simulink model "robot_adaptive_control"  (Simulink 7.2)
settings: Solver=ode45  StartTime=0.0  StopTime=20  RelTol=1e-3
libraries: dspmtrx3 x9, simulink x3
settings Model: Creator=GILL  LastModifiedBy=Dany
settings ConfigComp: Description=Design Verifier Custom Configuration Component  DVMaxProcessTime=600  DVDisplayUnsatisfiableObjectives=on  DVModelCoverageObjectives=MCDC  DVMaxTestCaseSteps=500  DVTestSuiteOptimization=CombinedObjectives  DVSaveHarnessModel=on  DVSaveReport=on

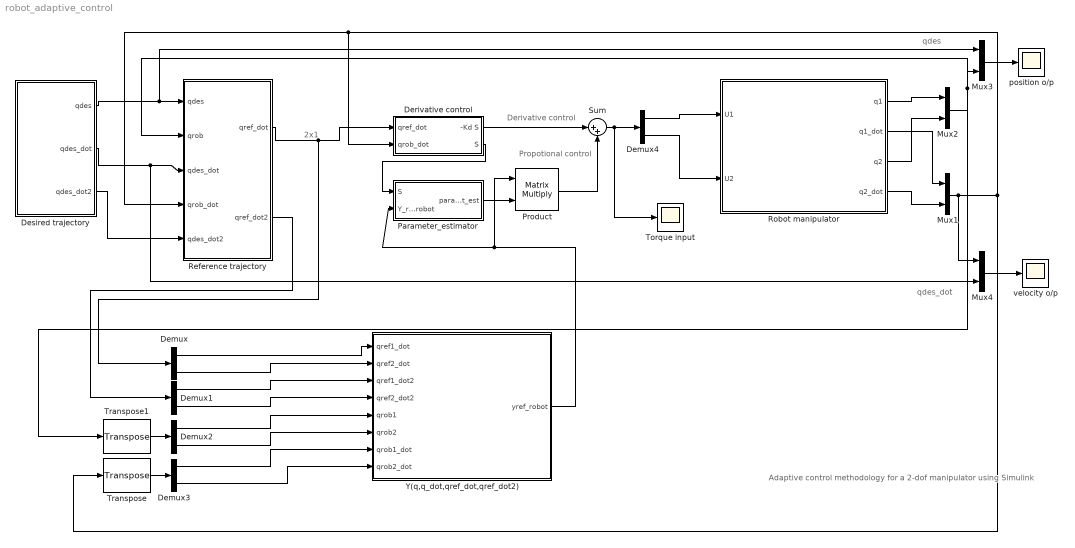
== system robot_adaptive_control ==
  note: 2x1
  note: qdes_dot
  note: qdes
  note: Propotional control
  note: Derivative control
  note: Adaptive control methodology for
      | a 2-dof manipulator using Simulink
  Demux{,1..4} (5 alike) : Demux  Outputs=2
  Derivative control : Subsystem
  Desired trajectory : Subsystem
  Mux{1..4} (4 alike) : Mux  Inputs=2
  Parameter_estimator : Subsystem
  Product : Product  Multiplication=Matrix(*)  OutDataType=fixdt(1, 16)  OutScaling=2^0  RndMeth=Zero
  Reference trajectory : Subsystem
  "Robot manipulator " : Subsystem
  Sum : Sum  Inputs=|++
  "Torque input " : Scope
      settings: YMin=-1.6  YMax=0.3  SaveName=ScopeData2
  Transpose : dspmtrx3/Transpose  SystemSampleTime=-1  Hermitian=off  overflowFlag=off
  Transpose1 : dspmtrx3/Transpose  SystemSampleTime=-1  Hermitian=off  overflowFlag=off
  Y(q,q_dot,qref_dot,qref_dot2) : Stateflow chart
  "position o/p " : Scope
      settings: YMin=-1.6  YMax=0.3
  velocity o/p : Scope
      settings: YMin=-1.6  YMax=0.3
  wires:
  Desired trajectory/1(qdes) -> Reference trajectory/1(qdes), Mux3/1
  Desired trajectory/2(qdes_dot) -> Reference trajectory/3(qdes_dot), Mux4/2
  Desired trajectory/3(qdes_dot2) -> Reference trajectory/5(qdes_dot2)
  Reference trajectory/1(qref_dot) -> Derivative control/1(qref_dot), Demux/1
  Demux/1 -> Y(q,q_dot,qref_dot,qref_dot2)/1(qref1_dot)
  Demux/2 -> Y(q,q_dot,qref_dot,qref_dot2)/2(qref2_dot)
  Demux1/1 -> Y(q,q_dot,qref_dot,qref_dot2)/3(qref1_dot2)
  Demux1/2 -> Y(q,q_dot,qref_dot,qref_dot2)/4(qref2_dot2)
  Demux2/1 -> Y(q,q_dot,qref_dot,qref_dot2)/5(qrob1)
  Demux2/2 -> Y(q,q_dot,qref_dot,qref_dot2)/6(qrob2)
  Demux3/1 -> Y(q,q_dot,qref_dot,qref_dot2)/7(qrob1_dot)
  Demux3/2 -> Y(q,q_dot,qref_dot,qref_dot2)/8(qrob2_dot)
  Reference trajectory/2(qref_dot2) -> Demux1/1
  Derivative control/1(-Kd S) -> Sum/1
  Derivative control/2(S) -> Parameter_estimator/1(S)
  Product/1 -> Sum/2
  Sum/1 -> Demux4/1, "Torque input "/1
  Mux1/1 -> Mux4/1, Transpose/1, Derivative control/2(qrob_dot), Reference trajectory/4(qrob_dot)
  Mux2/1 -> Mux3/2, Transpose1/1, Reference trajectory/2(qrob)
  Transpose1/1 -> Demux2/1
  Transpose/1 -> Demux3/1
  Y(q,q_dot,qref_dot,qref_dot2)/1(yref_robot) -> Product/1, Parameter_estimator/2(Y_ref_robot)
  Parameter_estimator/1(paramt_est) -> Product/2
  Mux3/1 -> "position o/p "/1
  Mux4/1 -> velocity o/p/1
  Demux4/1 -> "Robot manipulator "/1(U1)
  Demux4/2 -> "Robot manipulator "/2(U2)
  "Robot manipulator "/1(q1) -> Mux2/1
  "Robot manipulator "/3(q2) -> Mux2/2
  "Robot manipulator "/2(q1_dot) -> Mux1/1
  "Robot manipulator "/4(q2_dot) -> Mux1/2

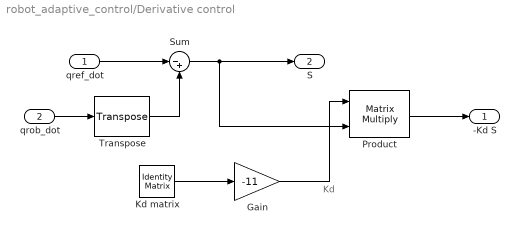
== system robot_adaptive_control/Derivative control ==
  note: Kd
  qref_dot : Inport
  qrob_dot : Inport  Port=2
  Gain : Gain  Gain=-11
  Kd matrix : dspmtrx3/Identity Matrix  Inherit=off  N=2  Ts=1  dataType=double  isSigned=on  wordLen=16  udDataType=sfix(16)  fracBitsMode=Best precision  numFracBits=15
  Product : Product  Multiplication=Matrix(*)  RndMeth=Zero
  Sum : Sum  Inputs=|-+
  Transpose : dspmtrx3/Transpose  SystemSampleTime=-1  Hermitian=off  overflowFlag=off
  -Kd S : Outport
  S : Outport  Port=2
  wires:
  qref_dot/1 -> Sum/1
  Sum/1 -> S/1, Product/2
  Kd matrix/1 -> Gain/1
  Product/1 -> -Kd S/1
  qrob_dot/1 -> Transpose/1
  Transpose/1 -> Sum/2
  Gain/1 -> Product/1

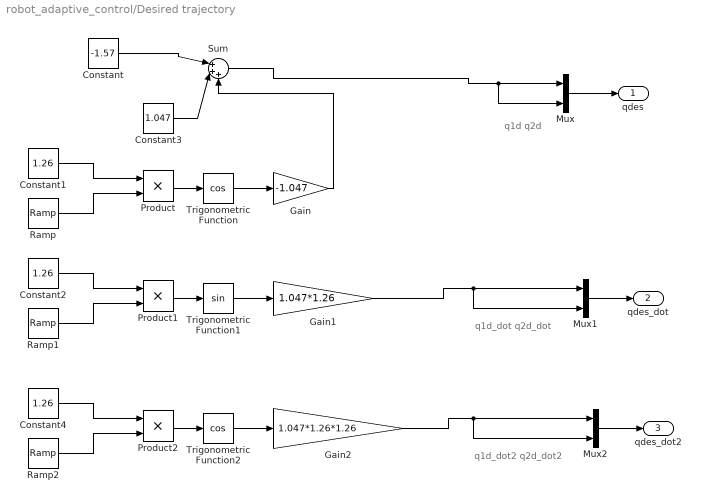
== system robot_adaptive_control/Desired trajectory ==
  note: q1d_dot
      | q2d_dot
  note: q1d
      | q2d
  note: q1d_dot2
      | q2d_dot2
  Constant : Constant  Value=-1.57
  Constant1 : Constant  Value=1.26
  Constant2 : Constant  Value=1.26
  Constant3 : Constant  Value=1.047
  Constant4 : Constant  Value=1.26
  Gain : Gain  Gain=-1.047
  Gain1 : Gain  Gain=1.047*1.26
  Gain2 : Gain  Gain=1.047*1.26*1.26
  Mux : Mux  Inputs=2
  Mux1 : Mux  Inputs=2
  Mux2 : Mux  Inputs=2
  Product : Product  RndMeth=Zero
  Product1 : Product  RndMeth=Zero
  Product2 : Product  RndMeth=Zero
  Ramp : simulink/Sources/Ramp  SystemSampleTime=-1  slope=1  start=0  X0=0
  Ramp1 : simulink/Sources/Ramp  SystemSampleTime=-1  slope=1  start=0  X0=0
  Ramp2 : simulink/Sources/Ramp  SystemSampleTime=-1  slope=1  start=0  X0=0
  Sum : Sum  Inputs=|+++
  Trigonometric Function : Trigonometry  Operator=cos
  Trigonometric Function1 : Trigonometry
  Trigonometric Function2 : Trigonometry  Operator=cos
  qdes : Outport
  qdes_dot : Outport  Port=2
  qdes_dot2 : Outport  Port=3
  wires:
  Constant/1 -> Sum/1
  Constant1/1 -> Product/1
  Constant3/1 -> Sum/2
  Ramp/1 -> Product/2
  Product/1 -> Trigonometric Function/1
  Trigonometric Function/1 -> Gain/1
  Gain/1 -> Sum/3
  Constant2/1 -> Product1/1
  Ramp1/1 -> Product1/2
  Product1/1 -> Trigonometric Function1/1
  Trigonometric Function1/1 -> Gain1/1
  Constant4/1 -> Product2/1
  Ramp2/1 -> Product2/2
  Product2/1 -> Trigonometric Function2/1
  Trigonometric Function2/1 -> Gain2/1
  Sum/1 -> Mux/1, Mux/2
  Mux/1 -> qdes/1
  Mux1/1 -> qdes_dot/1
  Gain1/1 -> Mux1/1, Mux1/2
  Mux2/1 -> qdes_dot2/1
  Gain2/1 -> Mux2/1, Mux2/2

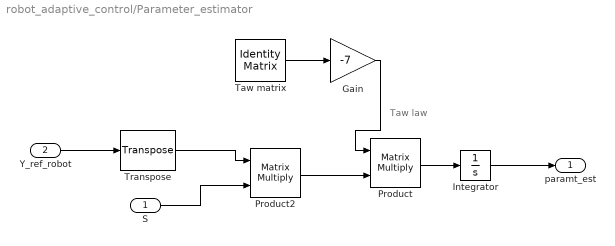
== system robot_adaptive_control/Parameter_estimator ==
  note: Taw law
  S : Inport  OutDataType=fixdt(1, 16)  OutScaling=2^0
  Y_ref_robot : Inport  Port=2  OutDataType=fixdt(1, 16)  OutScaling=2^0
  Gain : Gain  Gain=-7  ParameterDataType=fixdt(1, 16)  ParameterScaling=2^0  OutDataType=fixdt(1, 16)  OutScaling=2^0
  Integrator : Integrator
  Product : Product  Multiplication=Matrix(*)  OutDataType=fixdt(1, 16)  OutScaling=2^0  RndMeth=Zero
  Product2 : Product  Multiplication=Matrix(*)  OutDataType=fixdt(1, 16)  OutScaling=2^0  RndMeth=Zero
  Taw matrix : dspmtrx3/Identity Matrix  Inherit=off  N=5  Ts=1  dataType=double  isSigned=on  wordLen=16  udDataType=sfix(16)  fracBitsMode=Best precision  numFracBits=15
  Transpose : dspmtrx3/Transpose  SystemSampleTime=-1  Hermitian=off  overflowFlag=off
  paramt_est : Outport  OutDataType=fixdt(1, 16)  OutScaling=2^0
  wires:
  Product/1 -> Integrator/1
  Integrator/1 -> paramt_est/1
  Taw matrix/1 -> Gain/1
  Gain/1 -> Product/1
  Product2/1 -> Product/2
  Y_ref_robot/1 -> Transpose/1
  Transpose/1 -> Product2/1
  S/1 -> Product2/2

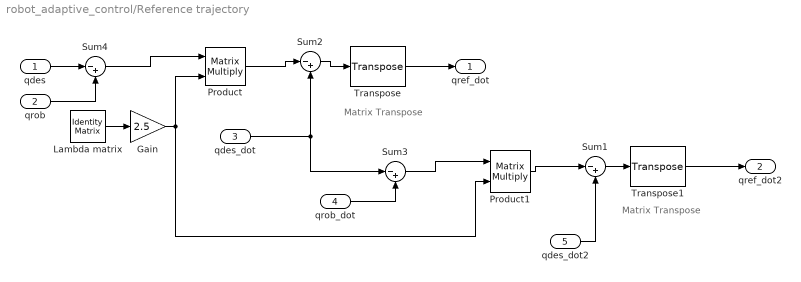
== system robot_adaptive_control/Reference trajectory ==
  note: Matrix Transpose
  note: Matrix Transpose
  qdes : Inport
  qrob : Inport  Port=2
  qdes_dot : Inport  Port=3
  qrob_dot : Inport  Port=4
  qdes_dot2 : Inport  Port=5
  Gain : Gain  Gain=2.5
  Lambda matrix : dspmtrx3/Identity Matrix  Inherit=off  N=2  Ts=1  dataType=double  isSigned=on  wordLen=16  udDataType=sfix(16)  fracBitsMode=Best precision  numFracBits=15
  Product : Product  Multiplication=Matrix(*)  RndMeth=Zero
  Product1 : Product  Multiplication=Matrix(*)  RndMeth=Zero
  Sum{1..4} (4 alike) : Sum  Inputs=|-+
  Transpose : dspmtrx3/Transpose  SystemSampleTime=-1  Hermitian=off  overflowFlag=off
  Transpose1 : dspmtrx3/Transpose  SystemSampleTime=-1  Hermitian=off  overflowFlag=off
  qref_dot : Outport
  qref_dot2 : Outport  Port=2
  wires:
  qdes/1 -> Sum4/1
  qrob/1 -> Sum4/2
  Sum4/1 -> Product/1
  Lambda matrix/1 -> Gain/1
  Gain/1 -> Product/2, Product1/2
  Product/1 -> Sum2/1
  qdes_dot/1 -> Sum2/2, Sum3/1
  qrob_dot/1 -> Sum3/2
  Sum3/1 -> Product1/1
  Product1/1 -> Sum1/1
  qdes_dot2/1 -> Sum1/2
  Transpose/1 -> qref_dot/1
  Sum2/1 -> Transpose/1
  Sum1/1 -> Transpose1/1
  Transpose1/1 -> qref_dot2/1

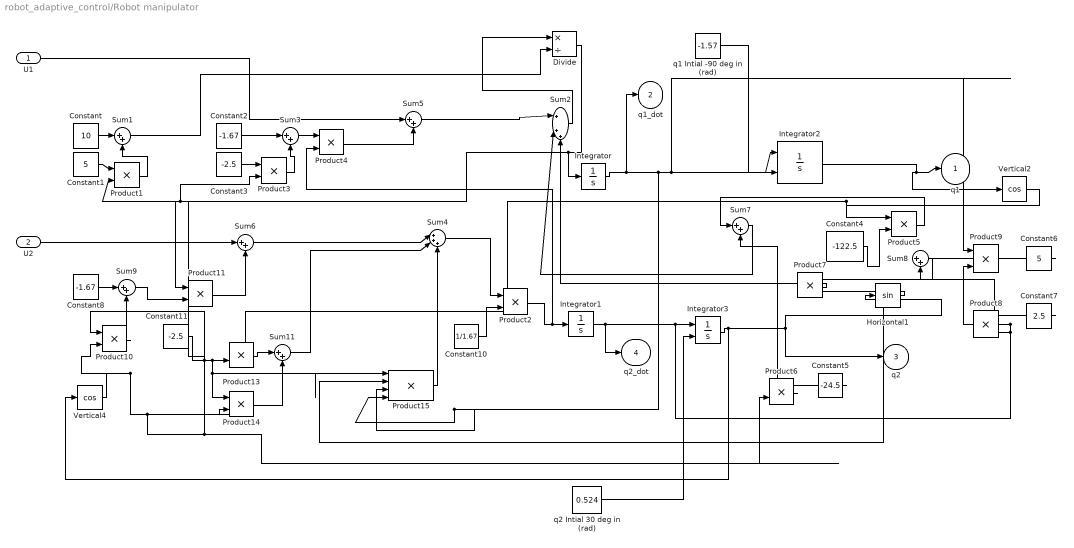
== system robot_adaptive_control/Robot manipulator  ==
  U1 : Inport
  U2 : Inport  Port=2
  Constant : Constant  Value=10
  Constant1 : Constant  Value=5
  Constant10 : Constant  Value=1/1.67
  Constant11 : Constant  Value=-2.5
  Constant2 : Constant  Value=-1.67
  Constant3 : Constant  Value=-2.5
  Constant4 : Constant  Value=-122.5
  Constant5 : Constant  Value=-24.5
  Constant6 : Constant  Value=5
  Constant7 : Constant  Value=2.5
  Constant8 : Constant  Value=-1.67
  Divide : Product  Inputs=*/
  Horizontal1 : Trigonometry
  Integrator : Integrator
  Integrator1 : Integrator
  Integrator2 : Integrator  InitialConditionSource=external
  Integrator3 : Integrator  InitialConditionSource=external
  Product{1..7,10..11,13..14} (11 alike) : Product  RndMeth=Zero
  Product15 : Product  Inputs=4  RndMeth=Zero
  Product8 : Product  Inputs=3  RndMeth=Zero
  Product9 : Product  Inputs=3  RndMeth=Zero
  Sum{1,3,5..9,11} (8 alike) : Sum  Inputs=|++
  Sum2 : Sum  Inputs=|+++
  Sum4 : Sum  Inputs=|+++
  Vertical2 : Trigonometry  Operator=cos
  Vertical4 : Trigonometry  Operator=cos
  q1 Intial -90 deg in (rad) : Constant  Value=-1.57
  q2 Intial 30 deg in (rad) : Constant  Value=0.524
  q1 : Outport
  q1_dot : Outport  Port=2
  q2 : Outport  Port=3
  q2_dot : Outport  Port=4
  wires:
  Integrator1/1 -> Integrator3/1, Product8/3, Product8/2, Product9/3, q2_dot/1
  Integrator3/1 -> Vertical4/1, Horizontal1/1, q2/1
  Integrator/1 -> Integrator2/1, Product9/1, Product15/3, Product15/4, q1_dot/1
  Integrator2/1 -> Vertical2/1, q1/1
  U1/1 -> Sum5/1
  Constant/1 -> Sum1/1
  Constant1/1 -> Product1/1
  Product1/1 -> Sum1/2
  Constant2/1 -> Sum3/1
  Constant3/1 -> Product3/1
  Product3/1 -> Sum3/2
  Sum3/1 -> Product4/1
  Vertical2/1 -> Product5/1, Product13/1
  Constant4/1 -> Product5/2
  Product5/1 -> Sum7/1
  Product6/1 -> Sum7/2
  Sum7/1 -> Sum2/2
  Horizontal1/1 -> Product7/2, Product15/2
  Constant6/1 -> Product9/2
  Constant7/1 -> Product8/1
  Product9/1 -> Sum8/1
  Product8/1 -> Sum8/2
  Sum8/1 -> Product7/1
  Product4/1 -> Sum5/2
  Product7/1 -> Sum2/3
  Sum5/1 -> Sum2/1
  U2/1 -> Sum6/1
  Constant8/1 -> Sum9/1
  Vertical4/1 -> Product14/2, Product6/2, Product1/2, Product3/2, Product10/2
  Product10/1 -> Sum9/2
  Sum9/1 -> Product11/2
  Product13/1 -> Sum11/1
  Product14/1 -> Sum11/2
  Constant5/1 -> Product6/1
  Constant11/1 -> Product13/2, Product14/1, Product15/1, Product10/1
  Sum11/1 -> Sum4/2
  Product15/1 -> Sum4/3
  Divide/1 -> Integrator/1, Product11/1
  Sum2/1 -> Divide/1
  Sum1/1 -> Divide/2
  Product2/1 -> Integrator1/1, Product4/2
  Sum4/1 -> Product2/1
  Constant10/1 -> Product2/2
  Product11/1 -> Sum6/2
  Sum6/1 -> Sum4/1
  q1 Intial -90 deg in (rad)/1 -> Integrator2/2
  q2 Intial 30 deg in (rad)/1 -> Integrator3/2

== matlab function Y(q,q_dot,qref_dot,qref_dot2) ==
  data: qref1_dot input double; yref_robot output double; qref2_dot input double; qref1_dot2 input double; qref2_dot2 input double; qrob1 input double; qrob2 input double; qrob1_dot input double; qrob2_dot input double
function yref_robot = fcn(qref1_dot,qref2_dot,qref1_dot2,qref2_dot2,qrob1,qrob2,qrob1_dot,qrob2_dot)
%#eml

yref_robot = [qref1_dot2+qref2_dot2, ( cos(qrob2)*(2*qref1_dot2 + qref2_dot2))-((sin(qrob2))*((qref1_dot*qrob2_dot)+(qref2_dot*qrob1_dot)+(qref2_dot*qrob2_dot))),qref1_dot2, 9.8* cos(qrob1), (9.8 * cos(qrob1+qrob2)) ;
    qref1_dot2+qref2_dot2, ((qref1_dot2 * cos(qrob2))+ (qrob1_dot * qref1_dot * sin(qrob2))), 0,0, cos(qrob1+qrob2)];
